simulink model "Simulink_Simulaiton"  (R2020a)
settings: Solver=ode23tb  StartTime=0.0  StopTime=10.0  RelTol=1e-3  EnableMultiTasking=on
undefined symbols (not defined in the file or in its folder): sigbuilder_block
libraries: powerlib x13, powerlib_meascontrol x2
settings Model: Creator=LENOVO  LastModifiedBy=x64
settings DataIOCC: LimitDataPoints=on  SaveFormat=Array  ReturnWorkspaceOutputs=off
settings OptimizationCC: LifeSpan=inf
settings DebuggingCC: SolverPrmCheckMsg=warning  SFUnexpectedBacktrackingDiag=warning  SFNoUnconditionalDefaultTransitionDiag=warning  SFExecutionAtInitializationDiag=none  ArithmeticOperatorsInVariantConditions=warning
settings HardwareCC: ProdBitPerPointer=32  ProdBitPerSizeT=32  ProdBitPerPtrDiffT=32  ProdLargestAtomicFloat=None  ProdIntDivRoundTo=Undefined  ProdEndianess=Unspecified  ProdWordSize=32  ProdHWDeviceType=32-bit Generic
settings ModelReferenceCC: PropagateSignalLabelsOutOfModel=off
settings SFSimCC: SimUseLocalCustomCode=off  CustomCodeUndefinedFunction=UseInterfaceOnly
settings RTWCC: RTWUseLocalCustomCode=off
settings CodeAppCC: StateflowObjectComments=on
settings GRTTargetCC: TargetLangStandard=C89/C90 (ANSI)
settings ConfigComp: CovMetricSettings=dw  CovHtmlReporting=on  CovSaveCumulativeToWorkspaceVar=on  CovSaveSingleToWorkspaceVar=on  CovExternalEMLEnable=off  CovSFcnEnable=off
settings SimscapeCC: SimscapeNormalizeSystem=off

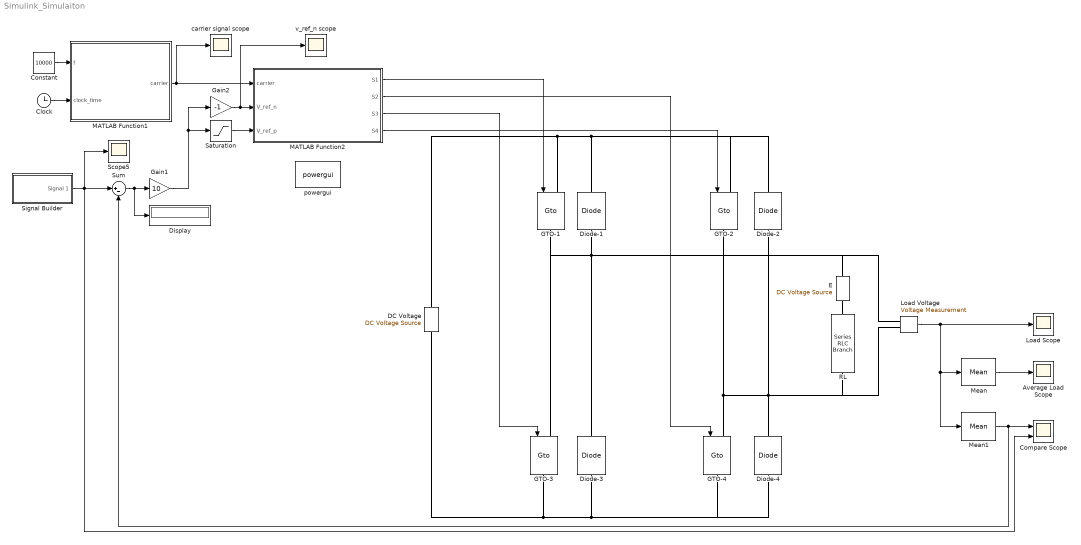
== system Simulink_Simulaiton ==
  " E" : powerlib/Electrical Sources/DC Voltage Source  Amplitude=50  Measurements=None
  Average Load Scope : Scope
  Clock : Clock
  Compare Scope : Scope  NumInputPorts=2
  Constant : Constant  Value=10000
  "DC Voltage " : powerlib/Electrical Sources/DC Voltage Source  Amplitude=270  Measurements=None
  Diode-{1..4} (4 alike) : powerlib/Power Electronics/Diode  Ron=0.001  Lon=0  Vf=0.8  IC=0  UseSnubber=off  Rs=500  Cs=250e-9  Measurements=off
  Display : Display
  GTO-{1..4} (4 alike) : powerlib/Power Electronics/Gto  Ron=0.01  Lon=0.00001  Vf=0.8  Tf=10e-6  Tt=20e-7  IC=0  Rs=10000  Cs=inf  Measurements=off
      settings: SourceProductBaseCode=PS
  Gain1 : Gain  Gain=10
  Gain2 : Gain  Gain=-1
  Load Scope : Scope
  Load Voltage : powerlib/Measurements/Voltage Measurement  PhasorSimulation=off  OutputType=Complex  PSBequivalent=0
  MATLAB Function1 : MATLAB Function  TreatAsAtomicUnit=on
  MATLAB Function2 : MATLAB Function  TreatAsAtomicUnit=on
  Mean : powerlib_meascontrol/Measurements/Mean  Freq=50  Vinit=0  Ts=0
  Mean1 : powerlib_meascontrol/Measurements/Mean  Freq=50  Vinit=0  Ts=0
  RL : powerlib/Elements/Series RLC Branch  LConnTagsString=__new0  RConnTagsString=__new0  BranchType=RL  Resistance=1  Inductance=1e-3  SetiL0=off  InitialCurrent=0  Capacitance=1e-6  Setx0=off  InitialVoltage=0  Measurements=None
  Saturation : Saturate  UpperLimit=1  LowerLimit=0
  Scope5 : Scope
  Signal Builder : Subsystem  Tag=STV Subsys  LoadFcn=sigbuilder_block('load');  StartFcn=sigbuilder_block('start');  StopFcn=sigbuilder_block('stop');  ClipboardFcn=sigbuilder_block('clipboard');  mask(Sigbuilder block){tuvar=[0:10]}
      mask help: Simulink:masks:SigbuilderBlock_MD
      mask init:
      | if ~strcmp(get_param(bdroot(gcbh),'SimulationStatus'),'stopped') tuvar = sigbuilder_block('maskInit'); end
      settings: CopyFcn=sigbuilder_block('copy');  DeleteFcn=sigbuilder_block('delete');  ModelCloseFcn=sigbuilder_block('modelClose');  PreSaveFcn=sigbuilder_block('preSave');  PauseFcn=sigbuilder_block('pause');  ContinueFcn=sigbuilder_block('continue');  NameChangeFcn=sigbuilder_block('namechange');  OpenFcn=sigbuilder_block('open',[0 30 1152 561.6 ]);  CloseFcn=sigbuilder_block('close');
      mask Display: plot(0, 0, 100, 100,[2, 2, 32, 32, 2], [68, 8, 8, 68, 68],[32, 2], [38, 38], [32, 19, 2],[53, 60, 44], [32, 17, 17, 2],[16, 16, 31, 31]);txt = getActiveGroup(gcbh);text(2, 100, txt,'verticalAlignment', 'top');
  Sum : Sum  Inputs=|+-
  carrier signal scope : Scope
  powergui : powerlib/powergui  Priority=1  SimulationMode=Discrete  SampleTime=1e-006  frequency=60  Iterations=50  frequencyindice=0  Pbase=100e6  ErrMax=1e-4  UnitsV=kV  UnitsW=MW  buscounter=0  FunctionMessages=off  echomessages=off  EnableUseOfTLC=off  CurrentSourceSwitches=off  DisableSnubberDevices=off  DisableRonSwitches=off  DisableVfSwitches=off  DisplayEquations=off  AutomaticDiscreteSolvers=off  SolverType=Tustin  Interpol=off  ExternalGateDelay=off  methode=off  Ts=100  x0status=blocks  SPID=off  SwTol=0  HookPort=off  NonlinearTolerance=1e-4  nMaxIteration=100  ContinueOnMaxIteration=off  RestoreLinks=warning  ResistiveCurrentMeasurement=off  Frange=[0:2:500]  Ylog=off  Xlog=on  ShowGrid=off  save=off  variable=ZData  structure=0  ZoomFFT=off  StartTime=0.0  cycles=1  DisplayStyle=1  fundamental=60  FreqAxis=off  MaxFrequency=1000  frequencyindicesteady=1  RmsSteady=1  display=off
  v_ref_n scope : Scope
  wires:
  Signal Builder/1(Signal 1) -> Compare Scope/2, Scope5/1, Sum/1
  Clock/1 -> MATLAB Function1/2(clock_time)
  Constant/1 -> MATLAB Function1/1(f)
  Sum/1 -> Display/1, Gain1/1
  Gain2/1 -> MATLAB Function2/2(V_ref_n), v_ref_n scope/1
  Gain1/1 -> Gain2/1, Saturation/1
  Load Voltage/1 -> Mean1/1, Mean/1, Load Scope/1
  Mean1/1 -> Compare Scope/1, Sum/2
  Saturation/1 -> MATLAB Function2/3(V_ref_p)
  Mean/1 -> Average Load Scope/1
  MATLAB Function1/1(carrier) -> MATLAB Function2/1(carrier), carrier signal scope/1
  MATLAB Function2/1(S1) -> GTO-1/1
  MATLAB Function2/2(S2) -> GTO-4/1
  MATLAB Function2/3(S3) -> GTO-3/1
  MATLAB Function2/4(S4) -> GTO-2/1
  connections:
  RL/LConn1 -- " E"/LConn1
  Diode-3/LConn1 -- GTO-3/RConn1 -- "DC Voltage "/LConn1 -- GTO-4/RConn1 -- Diode-4/LConn1
  "DC Voltage "/RConn1 -- Diode-2/RConn1 -- GTO-2/LConn1 -- Diode-1/RConn1 -- GTO-1/LConn1
  Diode-3/RConn1 -- Load Voltage/LConn1 -- " E"/RConn1 -- GTO-3/LConn1 -- GTO-1/RConn1 -- Diode-1/LConn1
  GTO-4/LConn1 -- RL/RConn1 -- Load Voltage/LConn2 -- Diode-4/RConn1 -- Diode-2/LConn1 -- GTO-2/RConn1

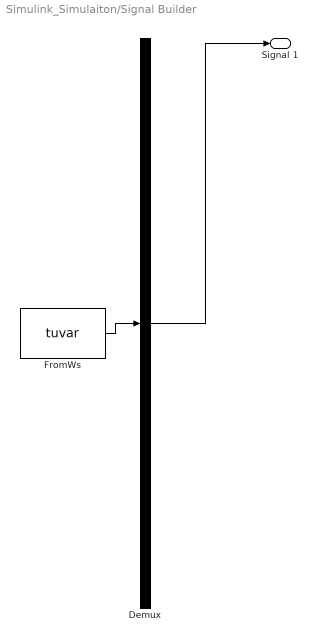
== system Simulink_Simulaiton/Signal Builder ==
  Demux : Demux  Tag=STV Demux  Outputs=1
      settings: DisplayOption=none
  FromWs : FromWorkspace  Tag=STV FromWs  VariableName=tuvar
      SigBuilderData=|
      | common.afterFinalStr = 'Extrapolate'
      | common.sampleTime = 0
      | dataSet.timeRange = [0 10]
      | dataSet.name = 'Group 1'
      | sbobj.Groups.Name = 'Group 1'
      | sbobj.Groups.Signals.Name = 'Signal 1'
      | sbobj.Groups.Signals.XData = [0 0.05 0.05 1 1.05 2 2 2.05 3 3.05 4 4 4.05 5 5.05 6 6 7 7.05 8 8 8.05 9 9.05 10]
      | sbobj.Groups.Signals.YData = [50 49.9 50 50 50 50 150 150 150 150 150 250 250 250 250 250 50 50 50 50 -150 -150 -150 -150 -150]
  Signal 1 : Outport  Tag=STV Outport
  wires:
  Demux/1 -> Signal 1/1
  FromWs/1 -> Demux/1

== matlab function Simulink_Simulaiton/MATLAB Function1 ==
  data: f input; carrier output; clock_time input
function carrier = Carrier_Generator(f, clock_time)
    %#codegen
    % Generates a triangular carrier wave for PWM
    % f: Frequency (Hz)
    % clock_time: Simulation time
    
    amplitude = 1;
    carrier = 0;
    multiplier = 1;
    
    half_period = 1/(2*f);              % p (Half period duration)
    peak_time = half_period/2;          % tepe_zaman (Time to reach peak)
    
    cycle_time = mod(clock_time, 2*half_period); % t (Current time in full cycle)
    local_time = mod(clock_time, half_period);   % zaman (Current time in half cycle)
    
    % Determine the polarity multiplier based on the cycle half
    if (cycle_time < half_period)
        multiplier = -1;
    else
        multiplier = 1;
    end
    
    % Generate the Triangle Shape
    if (local_time >= peak_time)
        % Falling edge calculation
        carrier = multiplier * ((amplitude/peak_time) * (half_period - local_time));
    else
        % Rising edge calculation
        carrier = multiplier * ((amplitude/peak_time) * local_time);
    end
    
    return
end

== matlab function Simulink_Simulaiton/MATLAB Function2 ==
  data: carrier input; V_ref_n input; V_ref_p input; S1 output; S2 output; S3 output; S4 output
function [S1, S2, S3, S4] = Unipolar_Gate_Logic(carrier, V_ref_n, V_ref_p)
    % Unipolar PWM Switching Logic Generation
    % carrier: Triangular carrier wave
    % V_ref_n: Negative reference control signal
    % V_ref_p: Positive reference control signal
    
    S1 = 0;
    S2 = 0;
    S3 = 0;
    S4 = 0;
    
    % Leg 1 Control (Controlled by V_ref_p)
    if (V_ref_p >= carrier)
        S1 = 1;  % Switch 1 ON
    end
    if (V_ref_p < carrier)
        S3 = 1;  % Switch 3 ON (Complementary to S1)
    end
    
    % Leg 2 Control (Controlled by V_ref_n)
    if (V_ref_n >= carrier)
        S4 = 1;  % Switch 4 ON
    end  
    if (V_ref_n < carrier)
        S2 = 1;  % Switch 2 ON (Complementary to S4)
    end
    
    return
end
